simulink library "halout"  (R2021b)
settings: Solver=VariableStepAuto  StartTime=0.0  StopTime=10.0  RelTol=1e-3
undefined symbols (not defined in the file): C_TASK_5MS_S, FALSE, KHAL_CAN1FDAPS3E2E_flg, KHAL_CAN1FDAPS3TxReq_flg, KHAL_CAN1FDVCU2E2E_flg, KHAL_CAN1FDVCU2TxReq_flg, KHAL_CAN1FDVCU3E2E_flg, KHAL_CAN1FDVCU3TxReq_flg, KHAL_CAN1TxReq_flg, KHAL_CAN2TxReq_flg, KHAL_CAN3FDVCU1TxReq_flg, KHAL_CAN3FDVCU2E2E_flg, KHAL_CAN3FDVCU2TxReq_flg, KHAL_CAN3TxReq_flg, KHAL_CAN4FDVCU1E2E_flg, KHAL_CAN4FDVCU1TxReq_flg, KHAL_CAN4TxReq_flg, KHAL_CAN5TxReq_flg, ONE_INT, TRUE, ZERO_INT
libraries: FVT_lib x383, simulink x179
(part 5 of 20)

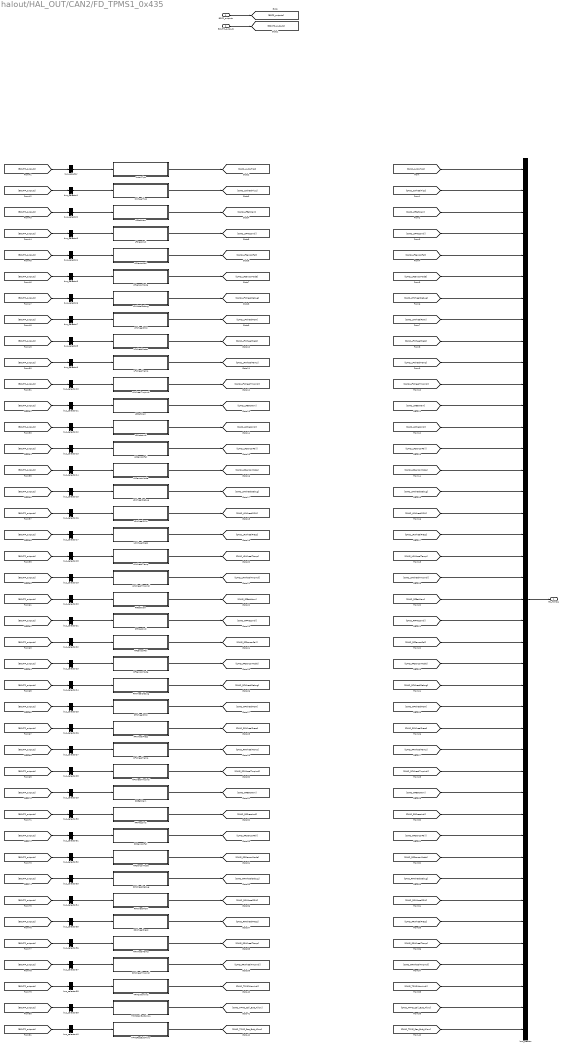
== system halout/HAL_OUT/CAN2/FD_TPMS1_0x435 ==
  BSCP_outputs : Inport  OutDataTypeStr=Bus: BSCP_outputs
  BOUTP_outputs : Inport  Port=2  OutDataTypeStr=Bus: BOUTP_outputs
  AutoLTips : Subsystem
  CWheelTips : Subsystem
  LFBatWarn : Subsystem
  LFPressIndi : Subsystem
  LFSensorFail : Subsystem
  LFSensorMode : Subsystem
  LFWheelDebug : Subsystem
  LFWheelPSW : Subsystem
  LFWheelPress : Subsystem
  LFWheelTemp : Subsystem
  LFWheelTmpIndi : Subsystem
  LRBatWarn : Subsystem
  LRPressIndi : Subsystem
  LRSensorFail : Subsystem
  LRSensorMode : Subsystem
  LRWheelDebug : Subsystem
  LRWheelPSW : Subsystem
  LRWheelPress : Subsystem
  LRWheelTemp : Subsystem
  LRWheelTmpIndi : Subsystem
  RFBatWarn : Subsystem
  RFPressIndi : Subsystem
  RFSensorFail : Subsystem
  RFSensorMode : Subsystem
  RFWheelDebug : Subsystem
  RFWheelPSW : Subsystem
  RFWheelPress : Subsystem
  RFWheelTemp : Subsystem
  RFWheelTmpIndi : Subsystem
  RRBatWarn : Subsystem
  RRPressIndi : Subsystem
  RRSensorFail : Subsystem
  RRSensorMode : Subsystem
  RRWheelDebug : Subsystem
  RRWheelPSW : Subsystem
  RRWheelPress : Subsystem
  RRWheelTemp : Subsystem
  RRWheelTmpIndi : Subsystem
  TPMSCaliButtAllow : Subsystem
  TPMSResButtAllow : Subsystem
  TPMSWarnIndi : Subsystem
  bus_creator : BusCreator  Inputs=41  OutDataTypeStr=Bus: DT_CAN2_SG_FD_TPMS1  NonVirtualBus=on
  bus_selector : BusSelector  OutputSignals=VOUTP_AutoLTips_enum
  bus_selector1 : BusSelector  OutputSignals=VOUTP_CWheelTips_enum
  bus_selector10 : BusSelector  OutputSignals=VOUTP_LFWheelTmpIndi_flg
  bus_selector11 : BusSelector  OutputSignals=VOUTP_LRBatWarn_flg
  bus_selector12 : BusSelector  OutputSignals=VOUTP_LRPressIndi_enum
  bus_selector13 : BusSelector  OutputSignals=VOUTP_LRSensorFail_flg
  bus_selector14 : BusSelector  OutputSignals=VOUTP_LRSensorMode_flg
  bus_selector15 : BusSelector  OutputSignals=VOUTP_LRWheelDebug_flg
  bus_selector16 : BusSelector  OutputSignals=VOUTP_LRWheelPSW_raw8
  bus_selector17 : BusSelector  OutputSignals=VOUTP_LRWheelPress_raw8
  bus_selector18 : BusSelector  OutputSignals=VOUTP_LRWheelTemp_C
  bus_selector19 : BusSelector  OutputSignals=VOUTP_LRWheelTmpIndi_flg
  bus_selector2 : BusSelector  OutputSignals=VOUTP_LFBatWarn_flg
  bus_selector20 : BusSelector  OutputSignals=VOUTP_RFBatWarn_flg
  bus_selector21 : BusSelector  OutputSignals=VOUTP_RFPressIndi_enum
  bus_selector22 : BusSelector  OutputSignals=VOUTP_RFSensorFail_flg
  bus_selector23 : BusSelector  OutputSignals=VOUTP_RFSensorMode_flg
  bus_selector24 : BusSelector  OutputSignals=VOUTP_RFWheelDebug_flg
  bus_selector25 : BusSelector  OutputSignals=VOUTP_RFWheelPSW_raw8
  bus_selector26 : BusSelector  OutputSignals=VOUTP_RFWheelPress_raw8
  bus_selector27 : BusSelector  OutputSignals=VOUTP_RFWheelTemp_C
  bus_selector28 : BusSelector  OutputSignals=VOUTP_RFWheelTmpIndi_flg
  bus_selector29 : BusSelector  OutputSignals=VOUTP_RRBatWarn_flg
  bus_selector3 : BusSelector  OutputSignals=VOUTP_LFPressIndi_enum
  bus_selector30 : BusSelector  OutputSignals=VOUTP_RRPressIndi_enum
  bus_selector31 : BusSelector  OutputSignals=VOUTP_RRSensorFail_flg
  bus_selector32 : BusSelector  OutputSignals=VOUTP_RRSensorMode_flg
  bus_selector33 : BusSelector  OutputSignals=VOUTP_RRWheelDebug_flg
  bus_selector34 : BusSelector  OutputSignals=VOUTP_RRWheelPSW_raw8
  bus_selector35 : BusSelector  OutputSignals=VOUTP_RRWheelPress_raw8
  bus_selector36 : BusSelector  OutputSignals=VOUTP_RRWheelTemp_C
  bus_selector37 : BusSelector  OutputSignals=VOUTP_RRWheelTmpIndi_flg
  bus_selector38 : BusSelector  OutputSignals=VOUTP_TPMSWarnIndi_enum
  bus_selector39 : BusSelector  OutputSignals=VOUTP_TPMSCaliButtAllow_flg
  bus_selector4 : BusSelector  OutputSignals=VOUTP_LFSensorFail_flg
  bus_selector40 : BusSelector  OutputSignals=VOUTP_TPMSResButtAllow_flg
  bus_selector5 : BusSelector  OutputSignals=VOUTP_LFSensorMode_flg
  bus_selector6 : BusSelector  OutputSignals=VOUTP_LFWheelDebug_flg
  bus_selector7 : BusSelector  OutputSignals=VOUTP_LFWheelPSW_raw8
  bus_selector8 : BusSelector  OutputSignals=VOUTP_LFWheelPress_raw8
  bus_selector9 : BusSelector  OutputSignals=VOUTP_LFWheelTemp_C
  FD_TPMS1 : Outport
  wires:
  BSCP_outputs/1 -> [BSCP_outputs]
  BOUTP_outputs/1 -> [BOUTP_outputs]
  [CAN2_AutoLTips] -> bus_creator/1  "CAN2_AutoLTips"
  [CAN2_CWheelTips] -> bus_creator/2  "CAN2_CWheelTips"
  [CAN2_LFBatWarn] -> bus_creator/3  "CAN2_LFBatWarn"
  [CAN2_LFPressIndi] -> bus_creator/4  "CAN2_LFPressIndi"
  [CAN2_LFSensorFail] -> bus_creator/5  "CAN2_LFSensorFail"
  [CAN2_LFSensorMode] -> bus_creator/6  "CAN2_LFSensorMode"
  [CAN2_LFWheelDebug] -> bus_creator/7  "CAN2_LFWheelDebug"
  [CAN2_LFWheelPSW] -> bus_creator/8  "CAN2_LFWheelPSW"
  [CAN2_LFWheelPress] -> bus_creator/9  "CAN2_LFWheelPress"
  [CAN2_LFWheelTemp] -> bus_creator/10  "CAN2_LFWheelTemp"
  [CAN2_LFWheelTmpIndi] -> bus_creator/11  "CAN2_LFWheelTmpIndi"
  [CAN2_LRBatWarn] -> bus_creator/12  "CAN2_LRBatWarn"
  [CAN2_LRPressIndi] -> bus_creator/13  "CAN2_LRPressIndi"
  [CAN2_LRSensorFail] -> bus_creator/14  "CAN2_LRSensorFail"
  [CAN2_LRSensorMode] -> bus_creator/15  "CAN2_LRSensorMode"
  [CAN2_LRWheelDebug] -> bus_creator/16  "CAN2_LRWheelDebug"
  [CAN2_LRWheelPSW] -> bus_creator/17  "CAN2_LRWheelPSW"
  [CAN2_LRWheelPress] -> bus_creator/18  "CAN2_LRWheelPress"
  [CAN2_LRWheelTemp] -> bus_creator/19  "CAN2_LRWheelTemp"
  [CAN2_LRWheelTmpIndi] -> bus_creator/20  "CAN2_LRWheelTmpIndi"
  [CAN2_RFBatWarn] -> bus_creator/21  "CAN2_RFBatWarn"
  [CAN2_RFPressIndi] -> bus_creator/22  "CAN2_RFPressIndi"
  [CAN2_RFSensorFail] -> bus_creator/23  "CAN2_RFSensorFail"
  [CAN2_RFSensorMode] -> bus_creator/24  "CAN2_RFSensorMode"
  [CAN2_RFWheelDebug] -> bus_creator/25  "CAN2_RFWheelDebug"
  [CAN2_RFWheelPSW] -> bus_creator/26  "CAN2_RFWheelPSW"
  [CAN2_RFWheelPress] -> bus_creator/27  "CAN2_RFWheelPress"
  [CAN2_RFWheelTemp] -> bus_creator/28  "CAN2_RFWheelTemp"
  [CAN2_RFWheelTmpIndi] -> bus_creator/29  "CAN2_RFWheelTmpIndi"
  [CAN2_RRBatWarn] -> bus_creator/30  "CAN2_RRBatWarn"
  [CAN2_RRPressIndi] -> bus_creator/31  "CAN2_RRPressIndi"
  [CAN2_RRSensorFail] -> bus_creator/32  "CAN2_RRSensorFail"
  [CAN2_RRSensorMode] -> bus_creator/33  "CAN2_RRSensorMode"
  [CAN2_RRWheelDebug] -> bus_creator/34  "CAN2_RRWheelDebug"
  [CAN2_RRWheelPSW] -> bus_creator/35  "CAN2_RRWheelPSW"
  [CAN2_RRWheelPress] -> bus_creator/36  "CAN2_RRWheelPress"
  [CAN2_RRWheelTemp] -> bus_creator/37  "CAN2_RRWheelTemp"
  [CAN2_RRWheelTmpIndi] -> bus_creator/38  "CAN2_RRWheelTmpIndi"
  [CAN2_TPMSWarnIndi] -> bus_creator/39  "CAN2_TPMSWarnIndi"
  [CAN2_TPMS_Cali_Butt_Allow] -> bus_creator/40  "CAN2_TPMS_Cali_Butt_Allow"
  [CAN2_TPMS_Res_Butt_Allow] -> bus_creator/41  "CAN2_TPMS_Res_Butt_Allow"
  bus_creator/1 -> FD_TPMS1/1
  AutoLTips/1(CAN2_AutoLTips) -> [CAN2_AutoLTips]
  CWheelTips/1(CAN2_CWheelTips) -> [CAN2_CWheelTips]
  LFBatWarn/1(CAN2_LFBatWarn) -> [CAN2_LFBatWarn]
  LFPressIndi/1(CAN2_LFPressIndi) -> [CAN2_LFPressIndi]
  LFSensorFail/1(CAN2_LFSensorFail) -> [CAN2_LFSensorFail]
  LFSensorMode/1(CAN2_LFSensorMode) -> [CAN2_LFSensorMode]
  LFWheelDebug/1(CAN2_LFWheelDebug) -> [CAN2_LFWheelDebug]
  LFWheelPSW/1(CAN2_LFWheelPSW) -> [CAN2_LFWheelPSW]
  LFWheelPress/1(CAN2_LFWheelPress) -> [CAN2_LFWheelPress]
  LFWheelTemp/1(CAN2_LFWheelTemp) -> [CAN2_LFWheelTemp]
  LFWheelTmpIndi/1(CAN2_LFWheelTmpIndi) -> [CAN2_LFWheelTmpIndi]
  LRBatWarn/1(CAN2_LRBatWarn) -> [CAN2_LRBatWarn]
  LRPressIndi/1(CAN2_LRPressIndi) -> [CAN2_LRPressIndi]
  LRSensorFail/1(CAN2_LRSensorFail) -> [CAN2_LRSensorFail]
  LRSensorMode/1(CAN2_LRSensorMode) -> [CAN2_LRSensorMode]
  LRWheelDebug/1(CAN2_LRWheelDebug) -> [CAN2_LRWheelDebug]
  LRWheelPSW/1(CAN2_LRWheelPSW) -> [CAN2_LRWheelPSW]
  LRWheelPress/1(CAN2_LRWheelPress) -> [CAN2_LRWheelPress]
  LRWheelTemp/1(CAN2_LRWheelTemp) -> [CAN2_LRWheelTemp]
  LRWheelTmpIndi/1(CAN2_LRWheelTmpIndi) -> [CAN2_LRWheelTmpIndi]
  RFBatWarn/1(CAN2_RFBatWarn) -> [CAN2_RFBatWarn]
  RFPressIndi/1(CAN2_RFPressIndi) -> [CAN2_RFPressIndi]
  RFSensorFail/1(CAN2_RFSensorFail) -> [CAN2_RFSensorFail]
  RFSensorMode/1(CAN2_RFSensorMode) -> [CAN2_RFSensorMode]
  RFWheelDebug/1(CAN2_RFWheelDebug) -> [CAN2_RFWheelDebug]
  RFWheelPSW/1(CAN2_RFWheelPSW) -> [CAN2_RFWheelPSW]
  RFWheelPress/1(CAN2_RFWheelPress) -> [CAN2_RFWheelPress]
  RFWheelTemp/1(CAN2_RFWheelTemp) -> [CAN2_RFWheelTemp]
  RFWheelTmpIndi/1(CAN2_RFWheelTmpIndi) -> [CAN2_RFWheelTmpIndi]
  RRBatWarn/1(CAN2_RRBatWarn) -> [CAN2_RRBatWarn]
  RRPressIndi/1(CAN2_RRPressIndi) -> [CAN2_RRPressIndi]
  RRSensorFail/1(CAN2_RRSensorFail) -> [CAN2_RRSensorFail]
  RRSensorMode/1(CAN2_RRSensorMode) -> [CAN2_RRSensorMode]
  RRWheelDebug/1(CAN2_RRWheelDebug) -> [CAN2_RRWheelDebug]
  RRWheelPSW/1(CAN2_RRWheelPSW) -> [CAN2_RRWheelPSW]
  RRWheelPress/1(CAN2_RRWheelPress) -> [CAN2_RRWheelPress]
  RRWheelTemp/1(CAN2_RRWheelTemp) -> [CAN2_RRWheelTemp]
  RRWheelTmpIndi/1(CAN2_RRWheelTmpIndi) -> [CAN2_RRWheelTmpIndi]
  TPMSWarnIndi/1(CAN2_TPMSWarnIndi) -> [CAN2_TPMSWarnIndi]
  TPMSCaliButtAllow/1(CAN2_TPMS_Cali_Butt_Allow) -> [CAN2_TPMS_Cali_Butt_Allow]
  TPMSResButtAllow/1(CAN2_TPMS_Res_Butt_Allow) -> [CAN2_TPMS_Res_Butt_Allow]
  bus_selector/1 -> AutoLTips/1(AutoLTips)  "<VOUTP_AutoLTips_enum>"
  [BOUTP_outputs] -> bus_selector/1
  bus_selector1/1 -> CWheelTips/1(CWheelTips)  "<VOUTP_CWheelTips_enum>"
  [BOUTP_outputs] -> bus_selector1/1
  bus_selector2/1 -> LFBatWarn/1(LFBatWarn)  "<VOUTP_LFBatWarn_flg>"
  [BOUTP_outputs] -> bus_selector2/1
  bus_selector3/1 -> LFPressIndi/1(LFPressIndi)  "<VOUTP_LFPressIndi_enum>"
  [BOUTP_outputs] -> bus_selector3/1
  bus_selector4/1 -> LFSensorFail/1(LFSensorFail)  "<VOUTP_LFSensorFail_flg>"
  [BOUTP_outputs] -> bus_selector4/1
  bus_selector5/1 -> LFSensorMode/1(LFSensorMode)  "<VOUTP_LFSensorMode_flg>"
  [BOUTP_outputs] -> bus_selector5/1
  bus_selector6/1 -> LFWheelDebug/1(LFWheelDebug)  "<VOUTP_LFWheelDebug_flg>"
  [BOUTP_outputs] -> bus_selector6/1
  bus_selector7/1 -> LFWheelPSW/1(LFWheelPSW)  "<VOUTP_LFWheelPSW_raw8>"
  [BOUTP_outputs] -> bus_selector7/1
  bus_selector8/1 -> LFWheelPress/1(LFWheelPress)  "<VOUTP_LFWheelPress_raw8>"
  [BOUTP_outputs] -> bus_selector8/1
  bus_selector9/1 -> LFWheelTemp/1(LFWheelTemp)  "<VOUTP_LFWheelTemp_C>"
  [BOUTP_outputs] -> bus_selector9/1
  bus_selector10/1 -> LFWheelTmpIndi/1(LFWheelTmpIndi)  "<VOUTP_LFWheelTmpIndi_flg>"
  [BOUTP_outputs] -> bus_selector10/1
  bus_selector11/1 -> LRBatWarn/1(LRBatWarn)  "<VOUTP_LRBatWarn_flg>"
  [BOUTP_outputs] -> bus_selector11/1
  bus_selector12/1 -> LRPressIndi/1(LRPressIndi)  "<VOUTP_LRPressIndi_enum>"
  [BOUTP_outputs] -> bus_selector12/1
  bus_selector13/1 -> LRSensorFail/1(LRSensorFail)  "<VOUTP_LRSensorFail_flg>"
  [BOUTP_outputs] -> bus_selector13/1
  bus_selector14/1 -> LRSensorMode/1(LRSensorMode)  "<VOUTP_LRSensorMode_flg>"
  [BOUTP_outputs] -> bus_selector14/1
  bus_selector15/1 -> LRWheelDebug/1(LRWheelDebug)  "<VOUTP_LRWheelDebug_flg>"
  [BOUTP_outputs] -> bus_selector15/1
  bus_selector16/1 -> LRWheelPSW/1(LRWheelPSW)  "<VOUTP_LRWheelPSW_raw8>"
  [BOUTP_outputs] -> bus_selector16/1
  bus_selector17/1 -> LRWheelPress/1(LRWheelPress)  "<VOUTP_LRWheelPress_raw8>"
  [BOUTP_outputs] -> bus_selector17/1
  bus_selector18/1 -> LRWheelTemp/1(LRWheelTemp)  "<VOUTP_LRWheelTemp_C>"
  [BOUTP_outputs] -> bus_selector18/1
  bus_selector19/1 -> LRWheelTmpIndi/1(LRWheelTmpIndi)  "<VOUTP_LRWheelTmpIndi_flg>"
  [BOUTP_outputs] -> bus_selector19/1
  bus_selector20/1 -> RFBatWarn/1(RFBatWarn)  "<VOUTP_RFBatWarn_flg>"
  [BOUTP_outputs] -> bus_selector20/1
  bus_selector21/1 -> RFPressIndi/1(RFPressIndi)  "<VOUTP_RFPressIndi_enum>"
  [BOUTP_outputs] -> bus_selector21/1
  bus_selector22/1 -> RFSensorFail/1(RFSensorFail)  "<VOUTP_RFSensorFail_flg>"
  [BOUTP_outputs] -> bus_selector22/1
  bus_selector23/1 -> RFSensorMode/1(RFSensorMode)  "<VOUTP_RFSensorMode_flg>"
  [BOUTP_outputs] -> bus_selector23/1
  bus_selector24/1 -> RFWheelDebug/1(RFWheelDebug)  "<VOUTP_RFWheelDebug_flg>"
  [BOUTP_outputs] -> bus_selector24/1
  bus_selector25/1 -> RFWheelPSW/1(RFWheelPSW)  "<VOUTP_RFWheelPSW_raw8>"
  [BOUTP_outputs] -> bus_selector25/1
  bus_selector26/1 -> RFWheelPress/1(RFWheelPress)  "<VOUTP_RFWheelPress_raw8>"
  [BOUTP_outputs] -> bus_selector26/1
  bus_selector27/1 -> RFWheelTemp/1(RFWheelTemp)  "<VOUTP_RFWheelTemp_C>"
  [BOUTP_outputs] -> bus_selector27/1
  bus_selector28/1 -> RFWheelTmpIndi/1(RFWheelTmpIndi)  "<VOUTP_RFWheelTmpIndi_flg>"
  [BOUTP_outputs] -> bus_selector28/1
  bus_selector29/1 -> RRBatWarn/1(RRBatWarn)  "<VOUTP_RRBatWarn_flg>"
  [BOUTP_outputs] -> bus_selector29/1
  bus_selector30/1 -> RRPressIndi/1(RRPressIndi)  "<VOUTP_RRPressIndi_enum>"
  [BOUTP_outputs] -> bus_selector30/1
  bus_selector31/1 -> RRSensorFail/1(RRSensorFail)  "<VOUTP_RRSensorFail_flg>"
  [BOUTP_outputs] -> bus_selector31/1
  bus_selector32/1 -> RRSensorMode/1(RRSensorMode)  "<VOUTP_RRSensorMode_flg>"
  [BOUTP_outputs] -> bus_selector32/1
  bus_selector33/1 -> RRWheelDebug/1(RRWheelDebug)  "<VOUTP_RRWheelDebug_flg>"
  [BOUTP_outputs] -> bus_selector33/1
  bus_selector34/1 -> RRWheelPSW/1(RRWheelPSW)  "<VOUTP_RRWheelPSW_raw8>"
  [BOUTP_outputs] -> bus_selector34/1
  bus_selector35/1 -> RRWheelPress/1(RRWheelPress)  "<VOUTP_RRWheelPress_raw8>"
  [BOUTP_outputs] -> bus_selector35/1
  bus_selector36/1 -> RRWheelTemp/1(RRWheelTemp)  "<VOUTP_RRWheelTemp_C>"
  [BOUTP_outputs] -> bus_selector36/1
  bus_selector37/1 -> RRWheelTmpIndi/1(RRWheelTmpIndi)  "<VOUTP_RRWheelTmpIndi_flg>"
  [BOUTP_outputs] -> bus_selector37/1
  bus_selector38/1 -> TPMSWarnIndi/1(TPMSWarnIndi)  "<VOUTP_TPMSWarnIndi_enum>"
  [BOUTP_outputs] -> bus_selector38/1
  bus_selector39/1 -> TPMSCaliButtAllow/1(TPMSCaliButtAllow)  "<VOUTP_TPMSCaliButtAllow_flg>"
  [BOUTP_outputs] -> bus_selector39/1
  bus_selector40/1 -> TPMSResButtAllow/1(TPMSResButtAllow)  "<VOUTP_TPMSResButtAllow_flg>"
  [BOUTP_outputs] -> bus_selector40/1

== system halout/HAL_OUT/CAN2/FD_TPMS2_0x436 ==
  BSCP_outputs : Inport  OutDataTypeStr=Bus: BSCP_outputs
  BOUTP_outputs : Inport  Port=2  OutDataTypeStr=Bus: BOUTP_outputs
  ID1ALTU : Subsystem
  ID1LocALTU : Subsystem
  ID1messageALTU : Subsystem
  ID2ALTU : Subsystem
  ID2LocALTU : Subsystem
  ID2messageALTU : Subsystem
  ID3ALTU : Subsystem
  ID3LocALTU : Subsystem
  ID3messageALTU : Subsystem
  ID4ALTU : Subsystem
  ID4LocALTU : Subsystem
  ID4messageALTU : Subsystem
  IDinALTU : Subsystem
  RFFATALTU : Subsystem
  S1WheelDebugALTU : Subsystem
  S2WheelDebugALTU : Subsystem
  S3WheelDebugALTU : Subsystem
  S4WheelDebugALTU : Subsystem
  bus_creator : BusCreator  Inputs=18  OutDataTypeStr=Bus: DT_CAN2_SG_FD_TPMS2  NonVirtualBus=on
  bus_selector : BusSelector  OutputSignals=VOUTP_S1ID_raw32
  bus_selector1 : BusSelector  OutputSignals=VOUTP_S1L_enum
  bus_selector10 : BusSelector  OutputSignals=VOUTP_S4L_enum
  bus_selector11 : BusSelector  OutputSignals=VOUTP_ID4messageALTU_raw8
  bus_selector12 : BusSelector  OutputSignals=VOUTP_IDin_raw32
  bus_selector13 : BusSelector  OutputSignals=VOUTP_FAT_flg
  bus_selector14 : BusSelector  OutputSignals=VOUTP_S1WheelDebugALTU_pct
  bus_selector15 : BusSelector  OutputSignals=VOUTP_S2WheelDebugALTU_pct
  bus_selector16 : BusSelector  OutputSignals=VOUTP_S3WheelDebugALTU_pct
  bus_selector17 : BusSelector  OutputSignals=VOUTP_S4WheelDebugALTU_pct
  bus_selector2 : BusSelector  OutputSignals=VOUTP_ID1messageALTU_raw8
  bus_selector3 : BusSelector  OutputSignals=VOUTP_S2ID_raw32
  bus_selector4 : BusSelector  OutputSignals=VOUTP_S2L_enum
  bus_selector5 : BusSelector  OutputSignals=VOUTP_ID2messageALTU_raw8
  bus_selector6 : BusSelector  OutputSignals=VOUTP_S3ID_raw32
  bus_selector7 : BusSelector  OutputSignals=VOUTP_S3L_enum
  bus_selector8 : BusSelector  OutputSignals=VOUTP_ID3messageALTU_raw8
  bus_selector9 : BusSelector  OutputSignals=VOUTP_S4ID_raw32
  FD_TPMS2 : Outport
  wires:
  BSCP_outputs/1 -> [BSCP_outputs]
  BOUTP_outputs/1 -> [BOUTP_outputs]
  [CAN2_ID1_ALTU] -> bus_creator/1  "CAN2_ID1_ALTU"
  [CAN2_ID1_Loc_ALTU] -> bus_creator/2  "CAN2_ID1_Loc_ALTU"
  [CAN2_ID1_message_ALTU] -> bus_creator/3  "CAN2_ID1_message_ALTU"
  [CAN2_ID2_ALTU] -> bus_creator/4  "CAN2_ID2_ALTU"
  [CAN2_ID2_Loc_ALTU] -> bus_creator/5  "CAN2_ID2_Loc_ALTU"
  [CAN2_ID2_message_ALTU] -> bus_creator/6  "CAN2_ID2_message_ALTU"
  [CAN2_ID3_ALTU] -> bus_creator/7  "CAN2_ID3_ALTU"
  [CAN2_ID3_Loc_ALTU] -> bus_creator/8  "CAN2_ID3_Loc_ALTU"
  [CAN2_ID3_message_ALTU] -> bus_creator/9  "CAN2_ID3_message_ALTU"
  [CAN2_ID4_ALTU] -> bus_creator/10  "CAN2_ID4_ALTU"
  [CAN2_ID4_Loc_ALTU] -> bus_creator/11  "CAN2_ID4_Loc_ALTU"
  [CAN2_ID4_message_ALTU] -> bus_creator/12  "CAN2_ID4_message_ALTU"
  [CAN2_IDin_ALTU] -> bus_creator/13  "CAN2_IDin_ALTU"
  [CAN2_RF_FAT_ALTU] -> bus_creator/14  "CAN2_RF_FAT_ALTU"
  [CAN2_S1WheelDebug_ALTU] -> bus_creator/15  "CAN2_S1WheelDebug_ALTU"
  [CAN2_S2WheelDebug_ALTU] -> bus_creator/16  "CAN2_S2WheelDebug_ALTU"
  [CAN2_S3WheelDebug_ALTU] -> bus_creator/17  "CAN2_S3WheelDebug_ALTU"
  [CAN2_S4WheelDebug_ALTU] -> bus_creator/18  "CAN2_S4WheelDebug_ALTU"
  bus_creator/1 -> FD_TPMS2/1
  ID1ALTU/1(CAN2_ID1_ALTU) -> [CAN2_ID1_ALTU]
  ID1LocALTU/1(CAN2_ID1_Loc_ALTU) -> [CAN2_ID1_Loc_ALTU]
  ID1messageALTU/1(CAN2_ID1_message_ALTU) -> [CAN2_ID1_message_ALTU]
  ID2ALTU/1(CAN2_ID2_ALTU) -> [CAN2_ID2_ALTU]
  ID2LocALTU/1(CAN2_ID2_Loc_ALTU) -> [CAN2_ID2_Loc_ALTU]
  ID2messageALTU/1(CAN2_ID2_message_ALTU) -> [CAN2_ID2_message_ALTU]
  ID3ALTU/1(CAN2_ID3_ALTU) -> [CAN2_ID3_ALTU]
  ID3LocALTU/1(CAN2_ID3_Loc_ALTU) -> [CAN2_ID3_Loc_ALTU]
  ID3messageALTU/1(CAN2_ID3_message_ALTU) -> [CAN2_ID3_message_ALTU]
  ID4ALTU/1(CAN2_ID4_ALTU) -> [CAN2_ID4_ALTU]
  ID4LocALTU/1(CAN2_ID4_Loc_ALTU) -> [CAN2_ID4_Loc_ALTU]
  ID4messageALTU/1(CAN2_ID4_message_ALTU) -> [CAN2_ID4_message_ALTU]
  IDinALTU/1(CAN2_IDin_ALTU) -> [CAN2_IDin_ALTU]
  RFFATALTU/1(CAN2_RF_FAT_ALTU) -> [CAN2_RF_FAT_ALTU]
  S1WheelDebugALTU/1(CAN2_S1WheelDebug_ALTU) -> [CAN2_S1WheelDebug_ALTU]
  S2WheelDebugALTU/1(CAN2_S2WheelDebug_ALTU) -> [CAN2_S2WheelDebug_ALTU]
  S3WheelDebugALTU/1(CAN2_S3WheelDebug_ALTU) -> [CAN2_S3WheelDebug_ALTU]
  S4WheelDebugALTU/1(CAN2_S4WheelDebug_ALTU) -> [CAN2_S4WheelDebug_ALTU]
  bus_selector/1 -> ID1ALTU/1(ID1ALTU)  "<VOUTP_S1ID_raw32>"
  [BOUTP_outputs] -> bus_selector/1
  bus_selector1/1 -> ID1LocALTU/1(ID1LocALTU)  "<VOUTP_S1L_enum>"
  [BOUTP_outputs] -> bus_selector1/1
  bus_selector2/1 -> ID1messageALTU/1(ID1messageALTU)  "<VOUTP_ID1messageALTU_raw8>"
  [BOUTP_outputs] -> bus_selector2/1
  bus_selector3/1 -> ID2ALTU/1(ID2ALTU)  "<VOUTP_S2ID_raw32>"
  [BOUTP_outputs] -> bus_selector3/1
  bus_selector4/1 -> ID2LocALTU/1(ID2LocALTU)  "<VOUTP_S2L_enum>"
  [BOUTP_outputs] -> bus_selector4/1
  bus_selector5/1 -> ID2messageALTU/1(ID2messageALTU)  "<VOUTP_ID2messageALTU_raw8>"
  [BOUTP_outputs] -> bus_selector5/1
  bus_selector6/1 -> ID3ALTU/1(ID3ALTU)  "<VOUTP_S3ID_raw32>"
  [BOUTP_outputs] -> bus_selector6/1
  bus_selector7/1 -> ID3LocALTU/1(ID3LocALTU)  "<VOUTP_S3L_enum>"
  [BOUTP_outputs] -> bus_selector7/1
  bus_selector8/1 -> ID3messageALTU/1(ID3messageALTU)  "<VOUTP_ID3messageALTU_raw8>"
  [BOUTP_outputs] -> bus_selector8/1
  bus_selector9/1 -> ID4ALTU/1(ID4ALTU)  "<VOUTP_S4ID_raw32>"
  [BOUTP_outputs] -> bus_selector9/1
  bus_selector10/1 -> ID4LocALTU/1(ID4LocALTU)  "<VOUTP_S4L_enum>"
  [BOUTP_outputs] -> bus_selector10/1
  bus_selector11/1 -> ID4messageALTU/1(ID4messageALTU)  "<VOUTP_ID4messageALTU_raw8>"
  [BOUTP_outputs] -> bus_selector11/1
  bus_selector12/1 -> IDinALTU/1(IDinALTU)  "<VOUTP_IDin_raw32>"
  [BOUTP_outputs] -> bus_selector12/1
  bus_selector13/1 -> RFFATALTU/1(RFFATALTU)  "<VOUTP_FAT_flg>"
  [BOUTP_outputs] -> bus_selector13/1
  bus_selector14/1 -> S1WheelDebugALTU/1(S1WheelDebugALTU)  "<VOUTP_S1WheelDebugALTU_pct>"
  [BOUTP_outputs] -> bus_selector14/1
  bus_selector15/1 -> S2WheelDebugALTU/1(S2WheelDebugALTU)  "<VOUTP_S2WheelDebugALTU_pct>"
  [BOUTP_outputs] -> bus_selector15/1
  bus_selector16/1 -> S3WheelDebugALTU/1(S3WheelDebugALTU)  "<VOUTP_S3WheelDebugALTU_pct>"
  [BOUTP_outputs] -> bus_selector16/1
  bus_selector17/1 -> S4WheelDebugALTU/1(S4WheelDebugALTU)  "<VOUTP_S4WheelDebugALTU_pct>"
  [BOUTP_outputs] -> bus_selector17/1

== system halout/HAL_OUT/CAN2/FD_V2L1_0x374 ==
  BSCP_outputs : Inport  OutDataTypeStr=Bus: BSCP_outputs
  BOUTP_outputs : Inport  Port=2  OutDataTypeStr=Bus: BOUTP_outputs
  Ground : Ground
  ReqOBCV2LEna : Subsystem
  ReqV2LIVIPopup : Subsystem
  ReqV2LSwOn : Subsystem
  bus_creator : BusCreator  Inputs=3  OutDataTypeStr=Bus: DT_CAN2_SG_FD_V2L1  NonVirtualBus=on
  bus_selector : BusSelector  OutputSignals=VOUTP_ReqOBCV2LEna_enum
  bus_selector1 : BusSelector  OutputSignals=VOUTP_ReqV2LIVIPopup_enum
  FD_V2L1 : Outport
  wires:
  BSCP_outputs/1 -> [BSCP_outputs]
  BOUTP_outputs/1 -> [BOUTP_outputs]
  [CAN2_Req_OBCV2LEna] -> bus_creator/1  "CAN2_Req_OBCV2LEna"
  [CAN2_Req_V2LSwOn] -> bus_creator/2  "CAN2_Req_V2LSwOn"
  [CAN2_Req_V2L_IVI_Popup] -> bus_creator/3  "CAN2_Req_V2L_IVI_Popup"
  bus_creator/1 -> FD_V2L1/1
  ReqOBCV2LEna/1(CAN2_Req_OBCV2LEna) -> [CAN2_Req_OBCV2LEna]
  ReqV2LSwOn/1(CAN2_Req_V2LSwOn) -> [CAN2_Req_V2LSwOn]
  ReqV2LIVIPopup/1(CAN2_Req_V2L_IVI_Popup) -> [CAN2_Req_V2L_IVI_Popup]
  bus_selector/1 -> ReqOBCV2LEna/1(ReqOBCV2LEna)  "<VOUTP_ReqOBCV2LEna_enum>"
  [BOUTP_outputs] -> bus_selector/1
  Ground/1 -> ReqV2LSwOn/1(ReqV2LSwOn)
  bus_selector1/1 -> ReqV2LIVIPopup/1(ReqV2LIVIPopup)  "<VOUTP_ReqV2LIVIPopup_enum>"
  [BOUTP_outputs] -> bus_selector1/1

== system halout/HAL_OUT/CAN2/FD_VCU0_0x1F0 ==
  BSCP_outputs : Inport  OutDataTypeStr=Bus: BSCP_outputs
  BOUTP_outputs : Inport  Port=2  OutDataTypeStr=Bus: BOUTP_outputs
  EVCCAplusPwrUpReq : Subsystem
  FDADC12VDetAvg : Subsystem
  FrTqSource : Subsystem
  Ground{,1..10} (11 alike) : Ground
  HVRlyOpFail : Subsystem
  HVTHCMSysAvail : Subsystem
  LVBattChrgtimeAct : Subsystem
  LVBattVoltSta : Subsystem
  LVChrgHoldTAct : Subsystem
  LVSilentChrgLv : Subsystem
  LVSilentChrgReq : Subsystem
  LVSilentChrgSta : Subsystem
  MCUActDisFail : Subsystem
  PMMAllowECUSleep : Subsystem
  PowerDownFault : Subsystem
  PowerDownState : Subsystem
  PowerUpFault : Subsystem
  PowerUpState : Subsystem
  PwrDownReq : Subsystem
  PwrStaConstraint : Subsystem
  PwrStaONTOIVIPopReq : Subsystem
  PwrStaONTOIVIPopT : Subsystem
  PwrStaSelect : Subsystem
  PwrStaTOSta : Subsystem
  PwrUpReq : Subsystem
  RrTqSource : Subsystem
  SchedChgTOSta : Subsystem
  SilentChkAllowSleep : Subsystem
  SysAllowReadySta : Subsystem
  SysPwrSta : Subsystem
  TCountSta : Subsystem
  TimerAllowSleep : Subsystem
  VCUBrkSWSta : Subsystem
  VCUFLDoorSta : Subsystem
  VCUFRDoorSta : Subsystem
  VCUHoodSWSta : Subsystem
  VCURLDoorSta : Subsystem
  VCURRDoorSta : Subsystem
  VCUTailgateSWSta : Subsystem
  VehHVPwrAvail4THCM : Subsystem
  bus_creator : BusCreator  Inputs=39  OutDataTypeStr=Bus: DT_CAN2_SG_FD_VCU0  NonVirtualBus=on
  bus_selector : BusSelector  OutputSignals=VOUTP_EvccAplusPwrUpReq_flg
  bus_selector1 : BusSelector  OutputSignals=VOUTP_FDADC12VDetAvg_mV
  bus_selector10 : BusSelector  OutputSignals=VOUTP_PMMAllowECUSleep_flg
  bus_selector11 : BusSelector  OutputSignals=VOUTP_PowerDownFault_enum
  bus_selector12 : BusSelector  OutputSignals=VOUTP_PowerDownState_enum
  bus_selector13 : BusSelector  OutputSignals=VOUTP_PowerUpFault_enum
  bus_selector14 : BusSelector  OutputSignals=VOUTP_PowerUpState_enum
  bus_selector15 : BusSelector  OutputSignals=VOUTP_PwrDownReq_enum
  bus_selector16 : BusSelector  OutputSignals=VOUTP_PwrStaConstraint_enum
  bus_selector17 : BusSelector  OutputSignals=VOUTP_PwrStaONTOPopReq_flg
  bus_selector18 : BusSelector  OutputSignals=VOUTP_IVIPwrStaONTOPopT_s
  bus_selector19 : BusSelector  OutputSignals=VOUTP_PwrStaSelect_enum
  bus_selector2 : BusSelector  OutputSignals=VOUTP_TqSourceFr_enum
  bus_selector20 : BusSelector  OutputSignals=VOUTP_PwrStaTOSta_enum
  bus_selector21 : BusSelector  OutputSignals=VOUTP_PwrUpReq_enum
  bus_selector22 : BusSelector  OutputSignals=VOUTP_TqSourceRr_enum
  bus_selector23 : BusSelector  OutputSignals=VOUTP_SilentChkAllowSleep_flg
  bus_selector24 : BusSelector  OutputSignals=VOUTP_SysPowerMode_enum
  bus_selector25 : BusSelector  OutputSignals=VOUTP_TCountSta_enum
  bus_selector26 : BusSelector  OutputSignals=VOUTP_TimerAllowSleep_flg
  bus_selector27 : BusSelector  OutputSignals=VOUTP_VehHVPwrAvail4THCM_W
  bus_selector3 : BusSelector  OutputSignals=VOUTP_HVTHCMSysAvail_enum
  bus_selector4 : BusSelector  OutputSignals=VOUTP_LVBattChrgTimeCnt_s
  bus_selector5 : BusSelector  OutputSignals=VOUTP_LVBattVoltSta_enum
  bus_selector6 : BusSelector  OutputSignals=VOUTP_LVChrgHoldTtimer_s
  bus_selector7 : BusSelector  OutputSignals=VOUTP_LVSilentChrgLv_enum
  bus_selector8 : BusSelector  OutputSignals=VOUTP_LVSilentChrgReq_flg
  bus_selector9 : BusSelector  OutputSignals=VOUTP_LVSilentChrgSta_enum
  FD_VCU0 : Outport
  wires:
  BSCP_outputs/1 -> [BSCP_outputs]
  BOUTP_outputs/1 -> [BOUTP_outputs]
  [CAN2_EVCCAplusPwrUpReq] -> bus_creator/1  "CAN2_EVCCAplusPwrUpReq"
  [CAN2_FDADC12VDetAvg] -> bus_creator/2  "CAN2_FDADC12VDetAvg"
  [CAN2_Fr_TqSource] -> bus_creator/3  "CAN2_Fr_TqSource"
  [CAN2_HVRlyOpFail] -> bus_creator/4  "CAN2_HVRlyOpFail"
  [CAN2_HVTHCMSysAvail] -> bus_creator/5  "CAN2_HVTHCMSysAvail"
  [CAN2_LVBattChrgtimeAct] -> bus_creator/6  "CAN2_LVBattChrgtimeAct"
  [CAN2_LVBattVoltSta] -> bus_creator/7  "CAN2_LVBattVoltSta"
  [CAN2_LVChrgHoldTAct] -> bus_creator/8  "CAN2_LVChrgHoldTAct"
  [CAN2_LVSilentChrgLv] -> bus_creator/9  "CAN2_LVSilentChrgLv"
  [CAN2_LVSilentChrgReq] -> bus_creator/10  "CAN2_LVSilentChrgReq"
  [CAN2_LVSilentChrgSta] -> bus_creator/11  "CAN2_LVSilentChrgSta"
  [CAN2_MCUActDisFail] -> bus_creator/12  "CAN2_MCUActDisFail"
  [CAN2_PMMAllowECUSleep] -> bus_creator/13  "CAN2_PMMAllowECUSleep"
  [CAN2_PowerDownFault] -> bus_creator/14  "CAN2_PowerDownFault"
  [CAN2_PowerDownState] -> bus_creator/15  "CAN2_PowerDownState"
  [CAN2_PowerUpFault] -> bus_creator/16  "CAN2_PowerUpFault"
  [CAN2_PowerUpState] -> bus_creator/17  "CAN2_PowerUpState"
  [CAN2_PwrDownReq] -> bus_creator/18  "CAN2_PwrDownReq"
  [CAN2_PwrStaConstraint] -> bus_creator/19  "CAN2_PwrStaConstraint"
  [CAN2_PwrStaONTOIVIPopReq] -> bus_creator/20  "CAN2_PwrStaONTOIVIPopReq"
  [CAN2_PwrStaONTOIVIPopT] -> bus_creator/21  "CAN2_PwrStaONTOIVIPopT"
  [CAN2_PwrStaSelect] -> bus_creator/22  "CAN2_PwrStaSelect"
  [CAN2_PwrStaTOSta] -> bus_creator/23  "CAN2_PwrStaTOSta"
  [CAN2_PwrUpReq] -> bus_creator/24  "CAN2_PwrUpReq"
  [CAN2_Rr_TqSource] -> bus_creator/25  "CAN2_Rr_TqSource"
  [CAN2_SchedChgTOSta] -> bus_creator/26  "CAN2_SchedChgTOSta"
  [CAN2_SilentChkAllowSleep] -> bus_creator/27  "CAN2_SilentChkAllowSleep"
  [CAN2_SysAllowReadySta] -> bus_creator/28  "CAN2_SysAllowReadySta"
  [CAN2_SysPwrSta] -> bus_creator/29  "CAN2_SysPwrSta"
  [CAN2_TCountSta] -> bus_creator/30  "CAN2_TCountSta"
  [CAN2_TimerAllowSleep] -> bus_creator/31  "CAN2_TimerAllowSleep"
  [CAN2_VCUBrkSWSta] -> bus_creator/32  "CAN2_VCUBrkSWSta"
  [CAN2_VCUFLDoorSta] -> bus_creator/33  "CAN2_VCUFLDoorSta"
  [CAN2_VCUFRDoorSta] -> bus_creator/34  "CAN2_VCUFRDoorSta"
  [CAN2_VCUHoodSWSta] -> bus_creator/35  "CAN2_VCUHoodSWSta"
  [CAN2_VCURLDoorSta] -> bus_creator/36  "CAN2_VCURLDoorSta"
  [CAN2_VCURRDoorSta] -> bus_creator/37  "CAN2_VCURRDoorSta"
  [CAN2_VCUTailgateSWSta] -> bus_creator/38  "CAN2_VCUTailgateSWSta"
  [CAN2_VehHVPwrAvail4THCM] -> bus_creator/39  "CAN2_VehHVPwrAvail4THCM"
  bus_creator/1 -> FD_VCU0/1
  EVCCAplusPwrUpReq/1(CAN2_EVCCAplusPwrUpReq) -> [CAN2_EVCCAplusPwrUpReq]
  FDADC12VDetAvg/1(CAN2_FDADC12VDetAvg) -> [CAN2_FDADC12VDetAvg]
  FrTqSource/1(CAN2_Fr_TqSource) -> [CAN2_Fr_TqSource]
  HVRlyOpFail/1(CAN2_HVRlyOpFail) -> [CAN2_HVRlyOpFail]
  HVTHCMSysAvail/1(CAN2_HVTHCMSysAvail) -> [CAN2_HVTHCMSysAvail]
  LVBattChrgtimeAct/1(CAN2_LVBattChrgtimeAct) -> [CAN2_LVBattChrgtimeAct]
  LVBattVoltSta/1(CAN2_LVBattVoltSta) -> [CAN2_LVBattVoltSta]
  LVChrgHoldTAct/1(CAN2_LVChrgHoldTAct) -> [CAN2_LVChrgHoldTAct]
  LVSilentChrgLv/1(CAN2_LVSilentChrgLv) -> [CAN2_LVSilentChrgLv]
  LVSilentChrgReq/1(CAN2_LVSilentChrgReq) -> [CAN2_LVSilentChrgReq]
  LVSilentChrgSta/1(CAN2_LVSilentChrgSta) -> [CAN2_LVSilentChrgSta]
  MCUActDisFail/1(CAN2_MCUActDisFail) -> [CAN2_MCUActDisFail]
  PMMAllowECUSleep/1(CAN2_PMMAllowECUSleep) -> [CAN2_PMMAllowECUSleep]
  PowerDownFault/1(CAN2_PowerDownFault) -> [CAN2_PowerDownFault]
  PowerDownState/1(CAN2_PowerDownState) -> [CAN2_PowerDownState]
  PowerUpFault/1(CAN2_PowerUpFault) -> [CAN2_PowerUpFault]
  PowerUpState/1(CAN2_PowerUpState) -> [CAN2_PowerUpState]
  PwrDownReq/1(CAN2_PwrDownReq) -> [CAN2_PwrDownReq]
  PwrStaConstraint/1(CAN2_PwrStaConstraint) -> [CAN2_PwrStaConstraint]
  PwrStaONTOIVIPopReq/1(CAN2_PwrStaONTOIVIPopReq) -> [CAN2_PwrStaONTOIVIPopReq]
  PwrStaONTOIVIPopT/1(CAN2_PwrStaONTOIVIPopT) -> [CAN2_PwrStaONTOIVIPopT]
  PwrStaSelect/1(CAN2_PwrStaSelect) -> [CAN2_PwrStaSelect]
  PwrStaTOSta/1(CAN2_PwrStaTOSta) -> [CAN2_PwrStaTOSta]
  PwrUpReq/1(CAN2_PwrUpReq) -> [CAN2_PwrUpReq]
  RrTqSource/1(CAN2_Rr_TqSource) -> [CAN2_Rr_TqSource]
  SchedChgTOSta/1(CAN2_SchedChgTOSta) -> [CAN2_SchedChgTOSta]
  SilentChkAllowSleep/1(CAN2_SilentChkAllowSleep) -> [CAN2_SilentChkAllowSleep]
  SysAllowReadySta/1(CAN2_SysAllowReadySta) -> [CAN2_SysAllowReadySta]
  SysPwrSta/1(CAN2_SysPwrSta) -> [CAN2_SysPwrSta]
  TCountSta/1(CAN2_TCountSta) -> [CAN2_TCountSta]
  TimerAllowSleep/1(CAN2_TimerAllowSleep) -> [CAN2_TimerAllowSleep]
  VCUBrkSWSta/1(CAN2_VCUBrkSWSta) -> [CAN2_VCUBrkSWSta]
  VCUFLDoorSta/1(CAN2_VCUFLDoorSta) -> [CAN2_VCUFLDoorSta]
  VCUFRDoorSta/1(CAN2_VCUFRDoorSta) -> [CAN2_VCUFRDoorSta]
  VCUHoodSWSta/1(CAN2_VCUHoodSWSta) -> [CAN2_VCUHoodSWSta]
  VCURLDoorSta/1(CAN2_VCURLDoorSta) -> [CAN2_VCURLDoorSta]
  VCURRDoorSta/1(CAN2_VCURRDoorSta) -> [CAN2_VCURRDoorSta]
  VCUTailgateSWSta/1(CAN2_VCUTailgateSWSta) -> [CAN2_VCUTailgateSWSta]
  VehHVPwrAvail4THCM/1(CAN2_VehHVPwrAvail4THCM) -> [CAN2_VehHVPwrAvail4THCM]
  bus_selector/1 -> EVCCAplusPwrUpReq/1(EVCCAplusPwrUpReq)  "<VOUTP_EvccAplusPwrUpReq_flg>"
  [BOUTP_outputs] -> bus_selector/1
  bus_selector1/1 -> FDADC12VDetAvg/1(FDADC12VDetAvg)  "<VOUTP_FDADC12VDetAvg_mV>"
  [BOUTP_outputs] -> bus_selector1/1
  bus_selector2/1 -> FrTqSource/1(FrTqSource)  "<VOUTP_TqSourceFr_enum>"
  [BOUTP_outputs] -> bus_selector2/1
  Ground/1 -> HVRlyOpFail/1(HVRlyOpFail)
  bus_selector3/1 -> HVTHCMSysAvail/1(HVTHCMSysAvail)  "<VOUTP_HVTHCMSysAvail_enum>"
  [BOUTP_outputs] -> bus_selector3/1
  bus_selector4/1 -> LVBattChrgtimeAct/1(LVBattChrgtimeAct)  "<VOUTP_LVBattChrgTimeCnt_s>"
  [BOUTP_outputs] -> bus_selector4/1
  bus_selector5/1 -> LVBattVoltSta/1(LVBattVoltSta)  "<VOUTP_LVBattVoltSta_enum>"
  [BOUTP_outputs] -> bus_selector5/1
  bus_selector6/1 -> LVChrgHoldTAct/1(LVChrgHoldTAct)  "<VOUTP_LVChrgHoldTtimer_s>"
  [BOUTP_outputs] -> bus_selector6/1
  bus_selector7/1 -> LVSilentChrgLv/1(LVSilentChrgLv)  "<VOUTP_LVSilentChrgLv_enum>"
  [BOUTP_outputs] -> bus_selector7/1
  bus_selector8/1 -> LVSilentChrgReq/1(LVSilentChrgReq)  "<VOUTP_LVSilentChrgReq_flg>"
  [BOUTP_outputs] -> bus_selector8/1
  bus_selector9/1 -> LVSilentChrgSta/1(LVSilentChrgSta)  "<VOUTP_LVSilentChrgSta_enum>"
  [BOUTP_outputs] -> bus_selector9/1
  Ground1/1 -> MCUActDisFail/1(MCUActDisFail)
  bus_selector10/1 -> PMMAllowECUSleep/1(PMMAllowECUSleep)  "<VOUTP_PMMAllowECUSleep_flg>"
  [BOUTP_outputs] -> bus_selector10/1
  bus_selector11/1 -> PowerDownFault/1(PowerDownFault)  "<VOUTP_PowerDownFault_enum>"
  [BOUTP_outputs] -> bus_selector11/1
  bus_selector12/1 -> PowerDownState/1(PowerDownState)  "<VOUTP_PowerDownState_enum>"
  [BOUTP_outputs] -> bus_selector12/1
  bus_selector13/1 -> PowerUpFault/1(PowerUpFault)  "<VOUTP_PowerUpFault_enum>"
  [BOUTP_outputs] -> bus_selector13/1
  bus_selector14/1 -> PowerUpState/1(PowerUpState)  "<VOUTP_PowerUpState_enum>"
  [BOUTP_outputs] -> bus_selector14/1
  bus_selector15/1 -> PwrDownReq/1(PwrDownReq)  "<VOUTP_PwrDownReq_enum>"
  [BOUTP_outputs] -> bus_selector15/1
  bus_selector16/1 -> PwrStaConstraint/1(PwrStaConstraint)  "<VOUTP_PwrStaConstraint_enum>"
  [BOUTP_outputs] -> bus_selector16/1
  bus_selector17/1 -> PwrStaONTOIVIPopReq/1(PwrStaONTOIVIPopReq)  "<VOUTP_PwrStaONTOPopReq_flg>"
  [BOUTP_outputs] -> bus_selector17/1
  bus_selector18/1 -> PwrStaONTOIVIPopT/1(PwrStaONTOIVIPopT)  "<VOUTP_IVIPwrStaONTOPopT_s>"
  [BOUTP_outputs] -> bus_selector18/1
  bus_selector19/1 -> PwrStaSelect/1(PwrStaSelect)  "<VOUTP_PwrStaSelect_enum>"
  [BOUTP_outputs] -> bus_selector19/1
  bus_selector20/1 -> PwrStaTOSta/1(PwrStaTOSta)  "<VOUTP_PwrStaTOSta_enum>"
  [BOUTP_outputs] -> bus_selector20/1
  bus_selector21/1 -> PwrUpReq/1(PwrUpReq)  "<VOUTP_PwrUpReq_enum>"
  [BOUTP_outputs] -> bus_selector21/1
  bus_selector22/1 -> RrTqSource/1(RrTqSource)  "<VOUTP_TqSourceRr_enum>"
  [BOUTP_outputs] -> bus_selector22/1
  Ground2/1 -> SchedChgTOSta/1(SchedChgTOSta)
  bus_selector23/1 -> SilentChkAllowSleep/1(SilentChkAllowSleep)  "<VOUTP_SilentChkAllowSleep_flg>"
  [BOUTP_outputs] -> bus_selector23/1
  Ground3/1 -> SysAllowReadySta/1(SysAllowReadySta)
  bus_selector24/1 -> SysPwrSta/1(SysPwrSta)  "<VOUTP_SysPowerMode_enum>"
  [BOUTP_outputs] -> bus_selector24/1
  bus_selector25/1 -> TCountSta/1(TCountSta)  "<VOUTP_TCountSta_enum>"
  [BOUTP_outputs] -> bus_selector25/1
  bus_selector26/1 -> TimerAllowSleep/1(TimerAllowSleep)  "<VOUTP_TimerAllowSleep_flg>"
  [BOUTP_outputs] -> bus_selector26/1
  Ground4/1 -> VCUBrkSWSta/1(VCUBrkSWSta)
  Ground5/1 -> VCUFLDoorSta/1(VCUFLDoorSta)
  Ground6/1 -> VCUFRDoorSta/1(VCUFRDoorSta)
  Ground7/1 -> VCUHoodSWSta/1(VCUHoodSWSta)
  Ground8/1 -> VCURLDoorSta/1(VCURLDoorSta)
  Ground9/1 -> VCURRDoorSta/1(VCURRDoorSta)
  Ground10/1 -> VCUTailgateSWSta/1(VCUTailgateSWSta)
  bus_selector27/1 -> VehHVPwrAvail4THCM/1(VehHVPwrAvail4THCM)  "<VOUTP_VehHVPwrAvail4THCM_W>"
  [BOUTP_outputs] -> bus_selector27/1

== system halout/HAL_OUT/CAN2/FD_VCU1_0x116 ==
  BSCP_outputs : Inport  OutDataTypeStr=Bus: BSCP_outputs
  BOUTP_outputs : Inport  Port=2  OutDataTypeStr=Bus: BOUTP_outputs
  ActiveDischReq : Subsystem
  CCCrlSta : Subsystem
  CSVCU1CAN2 : Subsystem
  CoastDwModeStaChk : Subsystem
  CreepSWSta : Subsystem
  DCDCEnaReq : Subsystem
  DCDCVoltSetpoint : Subsystem
  DemoModeStaChk : Subsystem
  DisengagePFail : Subsystem
  DrSeatSta : Subsystem
  DynoModeStaChk : Subsystem
  EngagePFail : Subsystem
  FDCVCUPwrSaveReqCmd : Subsystem
  FalseNPreventSta : Subsystem
  FrActvDmpDisabReq : Subsystem
  FrMCUEnaReq : Subsystem
  Ground{,1..8} (9 alike) : Ground
  HVBatCnctReq : Subsystem
  HVSysReadyToCharge : Subsystem
  LVChrgFuncStaChk : Subsystem
  MSACrlSta : Subsystem
  PrkReq : Subsystem
  PwrSta : Subsystem
  RCVCU1CAN2 : Subsystem
  RrActvDmpDisabReq : Subsystem
  RrMCUEnaReq : Subsystem
  ShiftGearPosn : Subsystem
  VCUOPDHold : Subsystem
  XWDMode : Subsystem
  bus_creator : BusCreator  Inputs=28  OutDataTypeStr=Bus: DT_CAN2_SG_FD_VCU1  NonVirtualBus=on
  bus_selector : BusSelector  OutputSignals=VOUTP_ActiveDischargeReq_flg
  bus_selector1 : BusSelector  OutputSignals=VOUTP_CCCtrlSta_enum
  bus_selector10 : BusSelector  OutputSignals=VOUTP_HVSysReadyToCharge_enum
  bus_selector11 : BusSelector  OutputSignals=VOUTP_MSACtrlSta_enum
  bus_selector12 : BusSelector  OutputSignals=VOUTP_ActParkRequest_flg
  bus_selector13 : BusSelector  OutputSignals=VOUTP_PowerSta_enum
  bus_selector14 : BusSelector  OutputSignals=VOUTP_RrActvDmpDisabReq_flg
  bus_selector15 : BusSelector  OutputSignals=VOUTP_RrMCUEnaReq_flg
  bus_selector16 : BusSelector  OutputSignals=VOUTP_ShiftGearPosn_enum
  bus_selector17 : BusSelector  OutputSignals=VOUTP_OPDHoldLamp_flg
  bus_selector18 : BusSelector  OutputSignals=VOUTP_DrivetrainSelect_enum
  bus_selector2 : BusSelector  OutputSignals=VOUTP_CreepON_flg
  bus_selector3 : BusSelector  OutputSignals=VOUTP_DCDCEnaReq_flg
  bus_selector4 : BusSelector  OutputSignals=VOUTP_DCDCVoltSetpoint_V
  bus_selector5 : BusSelector  OutputSignals=VOUTP_DrSeatSta_enum
  bus_selector6 : BusSelector  OutputSignals=VOUTP_DriveProtEn_flg
  bus_selector7 : BusSelector  OutputSignals=VOUTP_FrActvDmpDisabReq_flg
  bus_selector8 : BusSelector  OutputSignals=VOUTP_FrMCUEnaReq_flg
  bus_selector9 : BusSelector  OutputSignals=VOUTP_HVBatCnctReq_flg
  FD_VCU1 : Outport
  wires:
  BSCP_outputs/1 -> [BSCP_outputs]
  BOUTP_outputs/1 -> [BOUTP_outputs]
  [CAN2_ActiveDischReq] -> bus_creator/1  "CAN2_ActiveDischReq"
  [CAN2_CC_Crl_Sta] -> bus_creator/2  "CAN2_CC_Crl_Sta"
  [CAN2_CS_VCU1_CAN2] -> bus_creator/3  "CAN2_CS_VCU1_CAN2"
  [CAN2_CoastDwModeStaChk] -> bus_creator/4  "CAN2_CoastDwModeStaChk"
  [CAN2_CreepSW_Sta] -> bus_creator/5  "CAN2_CreepSW_Sta"
  [CAN2_DCDCEnaReq] -> bus_creator/6  "CAN2_DCDCEnaReq"
  [CAN2_DCDCVoltSetpoint] -> bus_creator/7  "CAN2_DCDCVoltSetpoint"
  [CAN2_DemoModeStaChk] -> bus_creator/8  "CAN2_DemoModeStaChk"
  [CAN2_DisengageP_Fail] -> bus_creator/9  "CAN2_DisengageP_Fail"
  [CAN2_Dr_SeatSta] -> bus_creator/10  "CAN2_Dr_SeatSta"
  [CAN2_DynoModeStaChk] -> bus_creator/11  "CAN2_DynoModeStaChk"
  [CAN2_EngageP_Fail] -> bus_creator/12  "CAN2_EngageP_Fail"
  [CAN2_FDC_VCU_PwrSaveReq_Cmd] -> bus_creator/13  "CAN2_FDC_VCU_PwrSaveReq_Cmd"
  [CAN2_FalseNPrevent_Sta] -> bus_creator/14  "CAN2_FalseNPrevent_Sta"
  [CAN2_Fr_ActvDmpDisabReq] -> bus_creator/15  "CAN2_Fr_ActvDmpDisabReq"
  [CAN2_Fr_MCUEnaReq] -> bus_creator/16  "CAN2_Fr_MCUEnaReq"
  [CAN2_HVBatCnctReq] -> bus_creator/17  "CAN2_HVBatCnctReq"
  [CAN2_HVSysReadyToCharge] -> bus_creator/18  "CAN2_HVSysReadyToCharge"
  [CAN2_LVChrgFuncStaChk] -> bus_creator/19  "CAN2_LVChrgFuncStaChk"
  [CAN2_MSA_Crl_Sta] -> bus_creator/20  "CAN2_MSA_Crl_Sta"
  [CAN2_PrkReq] -> bus_creator/21  "CAN2_PrkReq"
  [CAN2_PwrSta] -> bus_creator/22  "CAN2_PwrSta"
  [CAN2_RC_VCU1_CAN2] -> bus_creator/23  "CAN2_RC_VCU1_CAN2"
  [CAN2_Rr_ActvDmpDisabReq] -> bus_creator/24  "CAN2_Rr_ActvDmpDisabReq"
  [CAN2_Rr_MCUEnaReq] -> bus_creator/25  "CAN2_Rr_MCUEnaReq"
  [CAN2_ShiftGearPosn] -> bus_creator/26  "CAN2_ShiftGearPosn"
  [CAN2_VCU_OPDHold] -> bus_creator/27  "CAN2_VCU_OPDHold"
  [CAN2_XWDMode] -> bus_creator/28  "CAN2_XWDMode"
  bus_creator/1 -> FD_VCU1/1
  ActiveDischReq/1(CAN2_ActiveDischReq) -> [CAN2_ActiveDischReq]
  CCCrlSta/1(CAN2_CC_Crl_Sta) -> [CAN2_CC_Crl_Sta]
  CSVCU1CAN2/1(CAN2_CS_VCU1_CAN2) -> [CAN2_CS_VCU1_CAN2]
  CoastDwModeStaChk/1(CAN2_CoastDwModeStaChk) -> [CAN2_CoastDwModeStaChk]
  CreepSWSta/1(CAN2_CreepSW_Sta) -> [CAN2_CreepSW_Sta]
  DCDCEnaReq/1(CAN2_DCDCEnaReq) -> [CAN2_DCDCEnaReq]
  DCDCVoltSetpoint/1(CAN2_DCDCVoltSetpoint) -> [CAN2_DCDCVoltSetpoint]
  DemoModeStaChk/1(CAN2_DemoModeStaChk) -> [CAN2_DemoModeStaChk]
  DisengagePFail/1(CAN2_DisengageP_Fail) -> [CAN2_DisengageP_Fail]
  DrSeatSta/1(CAN2_Dr_SeatSta) -> [CAN2_Dr_SeatSta]
  DynoModeStaChk/1(CAN2_DynoModeStaChk) -> [CAN2_DynoModeStaChk]
  EngagePFail/1(CAN2_EngageP_Fail) -> [CAN2_EngageP_Fail]
  FDCVCUPwrSaveReqCmd/1(CAN2_FDC_VCU_PwrSaveReq_Cmd) -> [CAN2_FDC_VCU_PwrSaveReq_Cmd]
  FalseNPreventSta/1(CAN2_FalseNPrevent_Sta) -> [CAN2_FalseNPrevent_Sta]
  FrActvDmpDisabReq/1(CAN2_Fr_ActvDmpDisabReq) -> [CAN2_Fr_ActvDmpDisabReq]
  FrMCUEnaReq/1(CAN2_Fr_MCUEnaReq) -> [CAN2_Fr_MCUEnaReq]
  HVBatCnctReq/1(CAN2_HVBatCnctReq) -> [CAN2_HVBatCnctReq]
  HVSysReadyToCharge/1(CAN2_HVSysReadyToCharge) -> [CAN2_HVSysReadyToCharge]
  LVChrgFuncStaChk/1(CAN2_LVChrgFuncStaChk) -> [CAN2_LVChrgFuncStaChk]
  MSACrlSta/1(CAN2_MSA_Crl_Sta) -> [CAN2_MSA_Crl_Sta]
  PrkReq/1(CAN2_PrkReq) -> [CAN2_PrkReq]
  PwrSta/1(CAN2_PwrSta) -> [CAN2_PwrSta]
  RCVCU1CAN2/1(CAN2_RC_VCU1_CAN2) -> [CAN2_RC_VCU1_CAN2]
  RrActvDmpDisabReq/1(CAN2_Rr_ActvDmpDisabReq) -> [CAN2_Rr_ActvDmpDisabReq]
  RrMCUEnaReq/1(CAN2_Rr_MCUEnaReq) -> [CAN2_Rr_MCUEnaReq]
  ShiftGearPosn/1(CAN2_ShiftGearPosn) -> [CAN2_ShiftGearPosn]
  VCUOPDHold/1(CAN2_VCU_OPDHold) -> [CAN2_VCU_OPDHold]
  XWDMode/1(CAN2_XWDMode) -> [CAN2_XWDMode]
  bus_selector/1 -> ActiveDischReq/1(ActiveDischReq)  "<VOUTP_ActiveDischargeReq_flg>"
  [BOUTP_outputs] -> bus_selector/1
  bus_selector1/1 -> CCCrlSta/1(CCCrlSta)  "<VOUTP_CCCtrlSta_enum>"
  [BOUTP_outputs] -> bus_selector1/1
  Ground/1 -> CSVCU1CAN2/1(CSVCU1CAN2)
  Ground1/1 -> CoastDwModeStaChk/1(CoastDwModeStaChk)
  bus_selector2/1 -> CreepSWSta/1(CreepSWSta)  "<VOUTP_CreepON_flg>"
  [BOUTP_outputs] -> bus_selector2/1
  bus_selector3/1 -> DCDCEnaReq/1(DCDCEnaReq)  "<VOUTP_DCDCEnaReq_flg>"
  [BOUTP_outputs] -> bus_selector3/1
  bus_selector4/1 -> DCDCVoltSetpoint/1(DCDCVoltSetpoint)  "<VOUTP_DCDCVoltSetpoint_V>"
  [BOUTP_outputs] -> bus_selector4/1
  Ground2/1 -> DemoModeStaChk/1(DemoModeStaChk)
  Ground3/1 -> DisengagePFail/1(DisengagePFail)
  bus_selector5/1 -> DrSeatSta/1(DrSeatSta)  "<VOUTP_DrSeatSta_enum>"
  [BOUTP_outputs] -> bus_selector5/1
  Ground4/1 -> DynoModeStaChk/1(DynoModeStaChk)
  Ground5/1 -> EngagePFail/1(EngagePFail)
  Ground6/1 -> FDCVCUPwrSaveReqCmd/1(FDCVCUPwrSaveReqCmd)
  bus_selector6/1 -> FalseNPreventSta/1(FalseNPreventSta)  "<VOUTP_DriveProtEn_flg>"
  [BOUTP_outputs] -> bus_selector6/1
  bus_selector7/1 -> FrActvDmpDisabReq/1(FrActvDmpDisabReq)  "<VOUTP_FrActvDmpDisabReq_flg>"
  [BOUTP_outputs] -> bus_selector7/1
  bus_selector8/1 -> FrMCUEnaReq/1(FrMCUEnaReq)  "<VOUTP_FrMCUEnaReq_flg>"
  [BOUTP_outputs] -> bus_selector8/1
  bus_selector9/1 -> HVBatCnctReq/1(HVBatCnctReq)  "<VOUTP_HVBatCnctReq_flg>"
  [BOUTP_outputs] -> bus_selector9/1
  bus_selector10/1 -> HVSysReadyToCharge/1(HVSysReadyToCharge)  "<VOUTP_HVSysReadyToCharge_enum>"
  [BOUTP_outputs] -> bus_selector10/1
  Ground7/1 -> LVChrgFuncStaChk/1(LVChrgFuncStaChk)
  bus_selector11/1 -> MSACrlSta/1(MSACrlSta)  "<VOUTP_MSACtrlSta_enum>"
  [BOUTP_outputs] -> bus_selector11/1
  bus_selector12/1 -> PrkReq/1(PrkReq)  "<VOUTP_ActParkRequest_flg>"
  [BOUTP_outputs] -> bus_selector12/1
  bus_selector13/1 -> PwrSta/1(PwrSta)  "<VOUTP_PowerSta_enum>"
  [BOUTP_outputs] -> bus_selector13/1
  Ground8/1 -> RCVCU1CAN2/1(RCVCU1CAN2)
  bus_selector14/1 -> RrActvDmpDisabReq/1(RrActvDmpDisabReq)  "<VOUTP_RrActvDmpDisabReq_flg>"
  [BOUTP_outputs] -> bus_selector14/1
  bus_selector15/1 -> RrMCUEnaReq/1(RrMCUEnaReq)  "<VOUTP_RrMCUEnaReq_flg>"
  [BOUTP_outputs] -> bus_selector15/1
  bus_selector16/1 -> ShiftGearPosn/1(ShiftGearPosn)  "<VOUTP_ShiftGearPosn_enum>"
  [BOUTP_outputs] -> bus_selector16/1
  bus_selector17/1 -> VCUOPDHold/1(VCUOPDHold)  "<VOUTP_OPDHoldLamp_flg>"
  [BOUTP_outputs] -> bus_selector17/1
  bus_selector18/1 -> XWDMode/1(XWDMode)  "<VOUTP_DrivetrainSelect_enum>"
  [BOUTP_outputs] -> bus_selector18/1

== system halout/HAL_OUT/CAN2/FD_VCU2_0x154 ==
  BSCP_outputs : Inport  OutDataTypeStr=Bus: BSCP_outputs
  BOUTP_outputs : Inport  Port=2  OutDataTypeStr=Bus: BOUTP_outputs
  ACCCtrlAvail : Subsystem
  AccPedalOverride : Subsystem
  ActAPSPosn : Subsystem
  CSVCU2CAN1 : Subsystem
  DriverTq : Subsystem
  FrDriverTq : Subsystem
  Ground{,1..3} (4 alike) : Ground
  RCVCU2CAN1 : Subsystem
  RrDriverTq : Subsystem
  VehActPwr : Subsystem
  bus_creator : BusCreator  Inputs=9  OutDataTypeStr=Bus: DT_CAN2_SG_FD_VCU2  NonVirtualBus=on
  bus_selector : BusSelector  OutputSignals=VOUTP_ACCCtrlAvail_flg
  bus_selector1 : BusSelector  OutputSignals=VOUTP_ACCPedalOvrd_flg
  bus_selector2 : BusSelector  OutputSignals=VOUTP_ActAPSPosn_pct
  bus_selector3 : BusSelector  OutputSignals=VOUTP_DriverWhlTqDemFr_Nm
  bus_selector4 : BusSelector  OutputSignals=VOUTP_DriverWhlTqDemRr_Nm
  FD_VCU2 : Outport
  wires:
  BSCP_outputs/1 -> [BSCP_outputs]
  BOUTP_outputs/1 -> [BOUTP_outputs]
  [CAN2_ACC_CtrlAvail] -> bus_creator/1  "CAN2_ACC_CtrlAvail"
  [CAN2_AccPedal_Override] -> bus_creator/2  "CAN2_AccPedal_Override"
  [CAN2_ActAPSPosn] -> bus_creator/3  "CAN2_ActAPSPosn"
  [CAN2_CS_VCU2_CAN1] -> bus_creator/4  "CAN2_CS_VCU2_CAN1"
  [CAN2_DriverTq] -> bus_creator/5  "CAN2_DriverTq"
  [CAN2_Fr_DriverTq] -> bus_creator/6  "CAN2_Fr_DriverTq"
  [CAN2_RC_VCU2_CAN1] -> bus_creator/7  "CAN2_RC_VCU2_CAN1"
  [CAN2_Rr_DriverTq] -> bus_creator/8  "CAN2_Rr_DriverTq"
  [CAN2_VehActPwr] -> bus_creator/9  "CAN2_VehActPwr"
  bus_creator/1 -> FD_VCU2/1
  ACCCtrlAvail/1(CAN2_ACC_CtrlAvail) -> [CAN2_ACC_CtrlAvail]
  AccPedalOverride/1(CAN2_AccPedal_Override) -> [CAN2_AccPedal_Override]
  ActAPSPosn/1(CAN2_ActAPSPosn) -> [CAN2_ActAPSPosn]
  CSVCU2CAN1/1(CAN2_CS_VCU2_CAN1) -> [CAN2_CS_VCU2_CAN1]
  DriverTq/1(CAN2_DriverTq) -> [CAN2_DriverTq]
  FrDriverTq/1(CAN2_Fr_DriverTq) -> [CAN2_Fr_DriverTq]
  RCVCU2CAN1/1(CAN2_RC_VCU2_CAN1) -> [CAN2_RC_VCU2_CAN1]
  RrDriverTq/1(CAN2_Rr_DriverTq) -> [CAN2_Rr_DriverTq]
  VehActPwr/1(CAN2_VehActPwr) -> [CAN2_VehActPwr]
  bus_selector/1 -> ACCCtrlAvail/1(ACCCtrlAvail)  "<VOUTP_ACCCtrlAvail_flg>"
  [BOUTP_outputs] -> bus_selector/1
  bus_selector1/1 -> AccPedalOverride/1(AccPedalOverride)  "<VOUTP_ACCPedalOvrd_flg>"
  [BOUTP_outputs] -> bus_selector1/1
  bus_selector2/1 -> ActAPSPosn/1(ActAPSPosn)  "<VOUTP_ActAPSPosn_pct>"
  [BOUTP_outputs] -> bus_selector2/1
  Ground/1 -> CSVCU2CAN1/1(CSVCU2CAN1)
  Ground1/1 -> DriverTq/1(DriverTq)
  bus_selector3/1 -> FrDriverTq/1(FrDriverTq)  "<VOUTP_DriverWhlTqDemFr_Nm>"
  [BOUTP_outputs] -> bus_selector3/1
  Ground2/1 -> RCVCU2CAN1/1(RCVCU2CAN1)
  bus_selector4/1 -> RrDriverTq/1(RrDriverTq)  "<VOUTP_DriverWhlTqDemRr_Nm>"
  [BOUTP_outputs] -> bus_selector4/1
  Ground3/1 -> VehActPwr/1(VehActPwr)

== system halout/HAL_OUT/CAN2/FD_VCU4_0x3C0 ==
  BSCP_outputs : Inport  OutDataTypeStr=Bus: BSCP_outputs
  BOUTP_outputs : Inport  Port=2  OutDataTypeStr=Bus: BOUTP_outputs
  EVDriveMode : Subsystem
  EngAGSCloseSta : Subsystem
  EngActvDmpDisabSta : Subsystem
  EngCoastDwSta : Subsystem
  EngPwrLockSta : Subsystem
  Ground{,1..5} (6 alike) : Ground
  VCUACCErr : Subsystem
  VCUISAErr : Subsystem
  VehMalfunLevel : Subsystem
  ZoneDRSCPCommErr : Subsystem
  bus_creator : BusCreator  Inputs=9  OutDataTypeStr=Bus: DT_CAN2_SG_FD_VCU4  NonVirtualBus=on
  bus_selector : BusSelector  OutputSignals=VOUTP_EVDriveMode_enum
  bus_selector1 : BusSelector  OutputSignals=VOUTP_IVIPwrLockSta_enum
  bus_selector2 : BusSelector  OutputSignals=VOUTP_VehMalfunLevel_enum
  FD_VCU4 : Outport
  wires:
  BSCP_outputs/1 -> [BSCP_outputs]
  BOUTP_outputs/1 -> [BOUTP_outputs]
  [CAN2_EVDriveMode] -> bus_creator/1  "CAN2_EVDriveMode"
  [CAN2_Eng_AGSCloseSta] -> bus_creator/2  "CAN2_Eng_AGSCloseSta"
  [CAN2_Eng_ActvDmpDisabSta] -> bus_creator/3  "CAN2_Eng_ActvDmpDisabSta"
  [CAN2_Eng_CoastDwSta] -> bus_creator/4  "CAN2_Eng_CoastDwSta"
  [CAN2_Eng_PwrLockSta] -> bus_creator/5  "CAN2_Eng_PwrLockSta"
  [CAN2_VCU_ACCErr] -> bus_creator/6  "CAN2_VCU_ACCErr"
  [CAN2_VCU_ISAErr] -> bus_creator/7  "CAN2_VCU_ISAErr"
  [CAN2_VehMalfunLevel] -> bus_creator/8  "CAN2_VehMalfunLevel"
  [CAN2_ZoneDR_SCP_CommErr] -> bus_creator/9  "CAN2_ZoneDR_SCP_CommErr"
  bus_creator/1 -> FD_VCU4/1
  EVDriveMode/1(CAN2_EVDriveMode) -> [CAN2_EVDriveMode]
  EngAGSCloseSta/1(CAN2_Eng_AGSCloseSta) -> [CAN2_Eng_AGSCloseSta]
  EngActvDmpDisabSta/1(CAN2_Eng_ActvDmpDisabSta) -> [CAN2_Eng_ActvDmpDisabSta]
  EngCoastDwSta/1(CAN2_Eng_CoastDwSta) -> [CAN2_Eng_CoastDwSta]
  EngPwrLockSta/1(CAN2_Eng_PwrLockSta) -> [CAN2_Eng_PwrLockSta]
  VCUACCErr/1(CAN2_VCU_ACCErr) -> [CAN2_VCU_ACCErr]
  VCUISAErr/1(CAN2_VCU_ISAErr) -> [CAN2_VCU_ISAErr]
  VehMalfunLevel/1(CAN2_VehMalfunLevel) -> [CAN2_VehMalfunLevel]
  ZoneDRSCPCommErr/1(CAN2_ZoneDR_SCP_CommErr) -> [CAN2_ZoneDR_SCP_CommErr]
  bus_selector/1 -> EVDriveMode/1(EVDriveMode)  "<VOUTP_EVDriveMode_enum>"
  [BOUTP_outputs] -> bus_selector/1
  Ground/1 -> EngAGSCloseSta/1(EngAGSCloseSta)
  Ground1/1 -> EngActvDmpDisabSta/1(EngActvDmpDisabSta)
  Ground2/1 -> EngCoastDwSta/1(EngCoastDwSta)
  bus_selector1/1 -> EngPwrLockSta/1(EngPwrLockSta)  "<VOUTP_IVIPwrLockSta_enum>"
  [BOUTP_outputs] -> bus_selector1/1
  Ground3/1 -> VCUACCErr/1(VCUACCErr)
  Ground4/1 -> VCUISAErr/1(VCUISAErr)
  bus_selector2/1 -> VehMalfunLevel/1(VehMalfunLevel)  "<VOUTP_VehMalfunLevel_enum>"
  [BOUTP_outputs] -> bus_selector2/1
  Ground5/1 -> ZoneDRSCPCommErr/1(ZoneDRSCPCommErr)
